simulink model "UAV_sync_known_sim"  (R2018b)
settings: Solver=ode23tb  StartTime=0.0  StopTime=35
values from neighbouring files (symbols this model uses):
  C_rho = 1.225    [SC42120_UAV_Preconditions.m]
  D0 = [M0 0 0 0 0 0 ... (first row only)    [SC42120_UAV_Preconditions.m]
  D1 = [eye(3)*M1 zeros(3,3) ... (first row only)    [UAV_sync_known.m]    (also in UAV_sync_unknown.m; UAV_sync_unknown_gap.m)
  Derivative_gain_phi = 50    [SC42120_UAV_Preconditions.m]
  Derivative_gain_psi = 50    [SC42120_UAV_Preconditions.m]
  Derivative_gain_theta = 50    [SC42120_UAV_Preconditions.m]
  Derivative_gain_x = 50    [SC42120_UAV_Preconditions.m]
  Derivative_gain_y = 50    [SC42120_UAV_Preconditions.m]
  Derivative_gain_z = 50    [SC42120_UAV_Preconditions.m]
  G = 9.80665    [SC42120_UAV_Preconditions.m]
  g0 = [0;0;-M0*G;0;0;0]    [SC42120_UAV_Preconditions.m]
  g1 = [0;0;-M1*G;0;0;0]    [UAV_sync_known.m]    (also in UAV_sync_unknown.m; UAV_sync_unknown_gap.m)
  I0 = [0.02 0 -0.01 ... (first row only)    [SC42120_UAV_Preconditions.m]
  I1 = [0.1 0 -0.01 ... (first row only)    [UAV_sync_known.m]    (also in UAV_sync_unknown.m; UAV_sync_unknown_gap.m)
  InitWind = [0;0;0]    [SC42120_UAV_Preconditions.m]
  Kp = diag(P)    [SC42120_UAV_Preconditions.m]
  Kv = diag(V)    [SC42120_UAV_Preconditions.m]
  M0 = 10    [SC42120_UAV_Preconditions.m]
  M1 = 20    [UAV_sync_known.m]    (also in UAV_sync_unknown.m; UAV_sync_unknown_gap.m)
  Proportional_phi = 50    [SC42120_UAV_Preconditions.m]
  Proportional_psi = 50    [SC42120_UAV_Preconditions.m]
  Proportional_theta = 50    [SC42120_UAV_Preconditions.m]
  Proportional_x = 50    [SC42120_UAV_Preconditions.m]
  Proportional_y = 50    [SC42120_UAV_Preconditions.m]
  Proportional_z = 50    [SC42120_UAV_Preconditions.m]
undefined symbols (not defined in the file or in its folder): Aero, APlane, Bxl, C, Ctr, deg, DiscIntNeverNeededParam, F, Guid, Init, Light, MIL, Path, rad, s, Trim, Utility
libraries: aerolibconvert2 x37, simulink x15, dspsigops x7, aerolibasang x6, shared6dof x3, simulink_extras x3, sharedutil x2, aerolibadyn x1, aerolibtransform2 x1, aerolibwind2 x1
(part 3 of 6)

== system UAV_sync_known_sim/Node 0/VF Approach/AUTOPILOT/Low-level Controllers/Pitch controller ==
  PitchReference : Inport  Unit=deg
  EulerAngles : Inport  Port=2  Unit=deg
  AngularRates : Inport  Port=3  Unit=deg/s
  Scaler : Inport  Port=4
  1/Ctr.Roll.RLL2SRV_TCONST : Gain  Gain=1/Ctr.Roll.RLL2SRV_TCONST
  Angle Conversion1 : aerolibconvert2/Angle Conversion  IU=deg  OU=rad
  Angle Conversion5 : aerolibconvert2/Angle Conversion  IU=deg  OU=rad
  Coordination offset : Subsystem
  Pitch PID : Subsystem
  Rate limiter : Saturate  UpperLimit=Ctr.Pitch.PTCH2SRV_RMAX_UP  LowerLimit=-Ctr.Pitch.PTCH2SRV_RMAX_DN  LinearizeAsGain=off
  Saturation1 : Saturate  UpperLimit=80  LowerLimit=-80
  Selector1 : Selector  InputPortWidth=3  IndexOptions=Index vector (dialog)  Indices=2  OutputSizes=1
  Selector2 : Selector  InputPortWidth=3  IndexOptions=Index vector (dialog)  Indices=1  OutputSizes=1
  Selector3 : Selector  InputPortWidth=3  IndexOptions=Index vector (dialog)  Indices=1  OutputSizes=1
  Selector4 : Selector  InputPortWidth=3  IndexOptions=Index vector (dialog)  Indices=2  OutputSizes=1
  Sum : Sum  Inputs=++|
  Sum1 : Sum  Inputs=|+-
  TRASH : Subsystem  Commented=on
  ElevDemand : Outport
  wires:
  AngularRates/1 -> Selector1/1
  Selector2/1 -> Angle Conversion1/1  "roll_angle"
  EulerAngles/1 -> Selector3/1, Selector2/1, Selector4/1
  Selector1/1 -> Pitch PID/3(Meas_pitch_rate)  "pitch_rate"
  Selector4/1 -> Sum1/2, [pitch_ang]
  PitchReference/1 -> Sum1/1
  Sum/1 -> Pitch PID/1(DesRate)
  Selector3/1 -> Pitch PID/4(Meas_roll_angle)
  Scaler/1 -> Pitch PID/2(Scaler)
  Coordination offset/1(Pitch_rate_correction) -> Sum/1
  Sum1/1 -> 1/Ctr.Roll.RLL2SRV_TCONST/1
  1/Ctr.Roll.RLL2SRV_TCONST/1 -> Rate limiter/1
  Rate limiter/1 -> Sum/2
  [pitch_ang] -> Angle Conversion5/1
  Saturation1/1 -> Coordination offset/2(bank)
  [Va] -> Coordination offset/3(Va)
  Angle Conversion5/1 -> Coordination offset/1(pitch)
  Angle Conversion1/1 -> Saturation1/1
  Pitch PID/1(ElevDemand) -> ElevDemand/1

== system UAV_sync_known_sim/Node 0/VF Approach/AUTOPILOT/Low-level Controllers/Roll controller ==
  RollReference : Inport  Unit=deg
  Euler angles : Inport  Port=2  Unit=deg
  AngularRates : Inport  Port=3  Unit=deg/s
  Scaler : Inport  Port=4
  Discrete PID Controller : simulink/Continuous/PID Controller  Controller=PI  Form=Parallel  TimeDomain=Discrete-time  SampleTime=Ctr.TS  IntegratorMethod=Forward Euler  FilterMethod=Forward Euler  ControllerParametersSource=internal  P=1.28067056525733  I=0.869761866515897  D=0  UseFilter=on  N=100  TunerSelectOption=Transfer Function Based (PID Tuner App)  InitialConditionSource=internal  InitialConditionForIntegrator=0  InitialConditionForFilter=0  DifferentiatorICPrevScaledInput=0  ExternalReset=none  TrackingMode=off  Kt=1  LimitOutput=on  UpperSaturationLimit=Ctr.Roll.RLL2SRV_RMAX  LowerSaturationLimit=-Ctr.Roll.RLL2SRV_RMAX  LinearizeAsGain=off  AntiWindupMode=clamping  Kb=1  POutMin=[]  POutMax=[]  IOutMin=[]  IOutMax=[]  DOutMin=[]  DOutMax=[]  NOutMin=[]  NOutMax=[]  SumOutMin=[]  SumOutMax=[]  SaturationOutMin=[]  SaturationOutMax=[]  PParamMin=[]  PParamMax=[]  IParamMin=[]  IParamMax=[]  DParamMin=[]  DParamMax=[]  NParamMin=[]  NParamMax=[]  KbParamMin=[]  KbParamMax=[]  KtParamMin=[]  KtParamMax=[]  KbOutMin=[]  KbOutMax=[]  KtOutMin=[]  KtOutMax=[]  IntegratorOutMin=[]  IntegratorOutMax=[]  FilterOutMin=[]  FilterOutMax=[]  SumI1OutMin=[]  SumI1OutMax=[]  SumI2OutMin=[]  SumI2OutMax=[]  SumI3OutMin=[]  SumI3OutMax=[]  SumI4OutMin=[]  SumI4OutMax=[]  SumDOutMin=[]  SumDOutMax=[]  DifferentiatorOutMin=[]  DifferentiatorOutMax=[]  FilterDiffOutCoefMin=[]  FilterDiffOutCoefMax=[]  ReciprocalOutMin=[]  ReciprocalOutMax=[]  SumDenOutMin=[]  SumDenOutMax=[]  SumNumOutMin=[]  SumNumOutMax=[]  DivideOutMin=[]  DivideOutMax=[]  IntegratorContinuousStateAttributes=''  IntegratorStateMustResolveToSignalObject=off  IntegratorRTWStateStorageClass=Auto  FilterContinuousStateAttributes=''  FilterStateMustResolveToSignalObject=off  FilterRTWStateStorageClass=Auto  ParallelPVariant=InternalParameters  IdealPVariant=Disabled  IVariant=InternalParameters  DVariant=Disabled  IntegratorVariant=Discrete  SatVariant=Enabled  AWVariant=DiscClampingParallel  PCopyVariant=Disabled  TRVariant=Disabled  FdbkBlocksVariant=Forward  IdealPFdbkVariant=Disabled  SatFdbkVariant=Disabled  DerivativeFilterVariant=Disabled  NVariant=Disabled  NCopyVariant=Disabled_SignalSpec  FilterICVariant=Disabled  IntegratorICVariant=InternalICs  ExternalResetVariant=Disabled  TRSumVariant=Passthrough  SumFdbkVariant=Disabled  SumVariant=Sum_PI
  Manual Switch : ManualSwitch  CurrentSetting=0
  Manual Switch1 : ManualSwitch
  OMEGA : Gain  Gain=Ctr.Roll.OMEGA
  Roll Rate Controller : Subsystem
  Roll Rate Controller (simpl. continuous) : Subsystem  Commented=on
  "Scaler " : InportShadow  Port=4
  Scope : Scope  NumInputPorts=2
  Scope1 : Scope
  Selector : Selector  InputPortWidth=3  IndexOptions=Index vector (dialog)  Indices=1  OutputSizes=1
  Selector1 : Selector  InputPortWidth=3  IndexOptions=Index vector (dialog)  Indices=1  OutputSizes=1
  Sum : Sum  Inputs=|+-
  gainsrmax(deg/s) : Saturate  UpperLimit=Ctr.Roll.RLL2SRV_RMAX  LowerLimit=-Ctr.Roll.RLL2SRV_RMAX
  AilDemand : Outport  Unit=deg
  wires:
  RollReference/1 -> Scope/1, Sum/1
  Scaler/1 -> Roll Rate Controller/3(Scaler)  "m/s"
  AngularRates/1 -> Selector1/1
  Euler angles/1 -> Selector/1
  Sum/1 -> OMEGA/1, Discrete PID Controller/1, Scope1/1
  Selector1/1 -> Roll Rate Controller (simpl. continuous)/2(Roll rate), Roll Rate Controller/2(Roll Rate)  "roll_rate"
  Selector/1 -> Scope/2, Sum/2
  Manual Switch/1 -> Roll Rate Controller (simpl. continuous)/1(Roll Rate Error), Roll Rate Controller/1(Desidered rate)  "roll_rate_erorr [deg/s]"
  Manual Switch1/1 -> AilDemand/1
  Roll Rate Controller/1(Ail_dem) -> Manual Switch1/1
  "Scaler "/1 -> Roll Rate Controller (simpl. continuous)/3(Scaler)  "m/s"
  Roll Rate Controller (simpl. continuous)/1(AilDemand) -> Manual Switch1/2
  OMEGA/1 -> gainsrmax(deg/s)/1
  gainsrmax(deg/s)/1 -> Manual Switch/2  "roll_rate_erorr [deg/s]"
  Discrete PID Controller/1 -> Manual Switch/1

== system UAV_sync_known_sim/Node 0/VF Approach/AUTOPILOT/Low-level Controllers/Side-slip angle controller ==
  note: - Ctr.Yaw.YAW2SRV_SLIP enables side-slip angle control (disabled)
      | - Ctr.Yaw.YAW2SRV_DAMP enables the yaw angle damping (enabled)
  note: Roll Mixer = Aileron Rudder Interconnect (ARI). Disabled cause it creates an additional roll-yaw cross-coupling.
  note: Roll mixer
  Yaw_rate : Inport
  "Euler angles " : Inport  Port=2
  accel_y : Inport  Port=3
  Scaler : Inport  Port=4
  AilDemand : Inport  Port=5
  Angle Conversion : aerolibconvert2/Angle Conversion  IU=rad  OU=deg
  Coordination offset : Subsystem
  "Ctr.Yaw.KFF_RDDRMIX " : Gain  Gain=-1*Ctr.Yaw.KFF_RDDRMIX
  Ctr.Yaw.YAW2SRV_DAMP : Gain  Gain=Ctr.Yaw.YAW2SRV_DAMP
  Ctr.Yaw.YAW2SRV_INT : Gain  Gain=Ctr.Yaw.YAW2SRV_INT
  Ctr.Yaw.YAW2SRV_SLIP : Gain  Gain=Ctr.Yaw.YAW2SRV_SLIP+0.25
  Discrete-Time Integrator : DiscreteIntegrator  SampleTime=Ctr.TS  UpperSaturationLimit=deg2rad(15)  LowerSaturationLimit=deg2rad(-15)  ICPrevOutput=DiscIntNeverNeededParam  ICPrevScaledInput=DiscIntNeverNeededParam
  Gain4 : Gain  Gain=-1
  High-Pass Filter : Subsystem
  Math Function : Math  Operator=square  SaturateOnIntegerOverflow=on
  Product : Product
  Saturation : Saturate  UpperLimit=45  LowerLimit=-45
  Scope : Scope
  Scope1 : Scope
  Scope2 : Scope
  Selector1 : Selector  InputPortWidth=3  IndexOptions=Index vector (dialog)  Indices=1  OutputSizes=1
  Selector4 : Selector  InputPortWidth=3  IndexOptions=Index vector (dialog)  Indices=2  OutputSizes=1
  Selector5 : Selector  InputPortWidth=3  IndexOptions=Index vector (dialog)  Indices=3  OutputSizes=1
  Sum : Sum  Inputs=|+-
  Sum1 : Sum  Inputs=|+-
  Sum2 : Sum  Inputs=|+-
  Sum3 : Sum  Inputs=|++
  on/off : Gain
  RudderDemand : Outport
  wires:
  Ctr.Yaw.YAW2SRV_SLIP/1 -> Sum/1
  Yaw_rate/1 -> Selector5/1
  Sum1/1 -> High-Pass Filter/1(In)  "r_err"
  High-Pass Filter/1(Out) -> Scope2/1, Sum2/2, Sum/2
  Sum/1 -> Ctr.Yaw.YAW2SRV_INT/1
  Ctr.Yaw.YAW2SRV_INT/1 -> Discrete-Time Integrator/1
  Discrete-Time Integrator/1 -> Sum2/1
  Sum2/1 -> Ctr.Yaw.YAW2SRV_DAMP/1
  Ctr.Yaw.YAW2SRV_DAMP/1 -> Product/1
  Scaler/1 -> Math Function/1
  Math Function/1 -> Product/2
  Product/1 -> Gain4/1
  Selector5/1 -> Sum1/1
  Angle Conversion/1 -> Sum3/1
  Gain4/1 -> Angle Conversion/1
  Sum3/1 -> Saturation/1
  "Ctr.Yaw.KFF_RDDRMIX "/1 -> Sum3/2
  Saturation/1 -> on/off/1
  AilDemand/1 -> "Ctr.Yaw.KFF_RDDRMIX "/1
  "Euler angles "/1 -> Selector1/1
  Coordination offset/1(yaw_rate_correction) -> Sum1/2
  Selector1/1 -> Coordination offset/1(Bank)
  accel_y/1 -> Selector4/1
  Selector4/1 -> Ctr.Yaw.YAW2SRV_SLIP/1, Scope/1
  on/off/1 -> RudderDemand/1, Scope1/1

== system UAV_sync_known_sim/Node 0/VF Approach/AUTOPILOT/Navigation Controller/PID ==
  err : Inport
  scaler : Inport  Port=2
  20Hz filter : DiscreteTransferFcn  Numerator=Ctr.Hdg2Roll.lowpass.num  Denominator=Ctr.Hdg2Roll.lowpass.den  SampleTime=Ctr.TS
  Constant9 : Constant  Value=Ctr.TS
  Digital Clock : DigitalClock  SampleTime=Ctr.TS
  Discrete Transfer Fcn : DiscreteTransferFcn  Numerator=[1 -1]  Denominator=[Ctr.TS 0]  SampleTime=Ctr.TS
  Discrete Transfer Fcn1 : DiscreteTransferFcn  Numerator=Ctr.TS  Denominator=[1 -1]  SampleTime=Ctr.TS
  Discrete Transfer Fcn2 : DiscreteTransferFcn  Numerator=1  Denominator=[1 -1]  SampleTime=Ctr.TS
  Goto : Goto  Commented=on  GotoTag=deltaT
  IMAX : Saturate  UpperLimit=Ctr.Hdg2Roll.IMAX  LowerLimit=-Ctr.Hdg2Roll.IMAX
  K_D : Gain  Commented=on  Gain=Ctr.Hdg2Roll.NAV_ROLL_D
  K_I : Gain  Gain=Ctr.Hdg2Roll.NAV_ROLL_I
  K_I1 : Gain  Gain=Ctr.Hdg2Roll.NAV_ROLL_I
  K_P : Gain  Gain=Ctr.Hdg2Roll.NAV_ROLL_P
  Manual Switch : ManualSwitch  CurrentSetting=0
  Product : Product
  Product2 : Product  Inputs=**
  Product3 : Product  Commented=on  Inputs=*/
  Product4 : Product
  Product5 : Product
  Scope : Scope  NumInputPorts=3
  Scope1 : Scope
  Scope2 : Scope  NumInputPorts=2
  Sum1 : Sum  Inputs=+++
  Sum3 : Sum  Commented=on  Inputs=|+-
  Sum4 : Sum  Inputs=|+-
  Unit Delay : UnitDelay  SampleTime=-1
  Unit Delay2 : UnitDelay  Commented=on  SampleTime=-1
  out : Outport
  wires:
  K_P/1 -> Product5/1
  err/1 -> Product/2, K_P/1, K_D/1, K_I/1
  IMAX/1 -> Scope/2, Sum1/2
  K_I/1 -> Discrete Transfer Fcn1/1
  Unit Delay/1 -> Sum4/2
  Digital Clock/1 -> Unit Delay/1, Sum4/1
  Manual Switch/1 -> Goto/1
  Constant9/1 -> Manual Switch/1
  Product2/1 -> IMAX/1
  20Hz filter/1 -> Product4/2
  Product4/1 -> Scope/3, Sum1/3
  Product5/1 -> Scope/1, Sum1/1
  Discrete Transfer Fcn1/1 -> Scope2/2, Product2/1
  scaler/1 -> Product2/2, Product5/2, Product4/1
  Sum1/1 -> out/1, Scope1/1
  K_D/1 -> Discrete Transfer Fcn/1
  Unit Delay2/1 -> Sum3/2
  Sum3/1 -> Product3/1
  Discrete Transfer Fcn/1 -> 20Hz filter/1
  Sum4/1 -> Product/1, Manual Switch/2
  K_I1/1 -> Discrete Transfer Fcn2/1
  Discrete Transfer Fcn2/1 -> Scope2/1
  Product/1 -> K_I1/1

== system UAV_sync_known_sim/Node 0/VF Approach/AUTOPILOT/Navigation Controller/Unwrap ==
  In : Inport
  Degrees to Radians : simulink_extras/Transformations/Degrees to Radians
  Radians to Degrees : simulink_extras/Transformations/Radians to Degrees
  Unwrap2 : dspsigops/Unwrap  tol=pi  InputProcessing=Columns as channels (frame based)  running=off
  Out : Outport
  wires:
  Unwrap2/1 -> Radians to Degrees/1
  In/1 -> Degrees to Radians/1
  Degrees to Radians/1 -> Unwrap2/1
  Radians to Degrees/1 -> Out/1

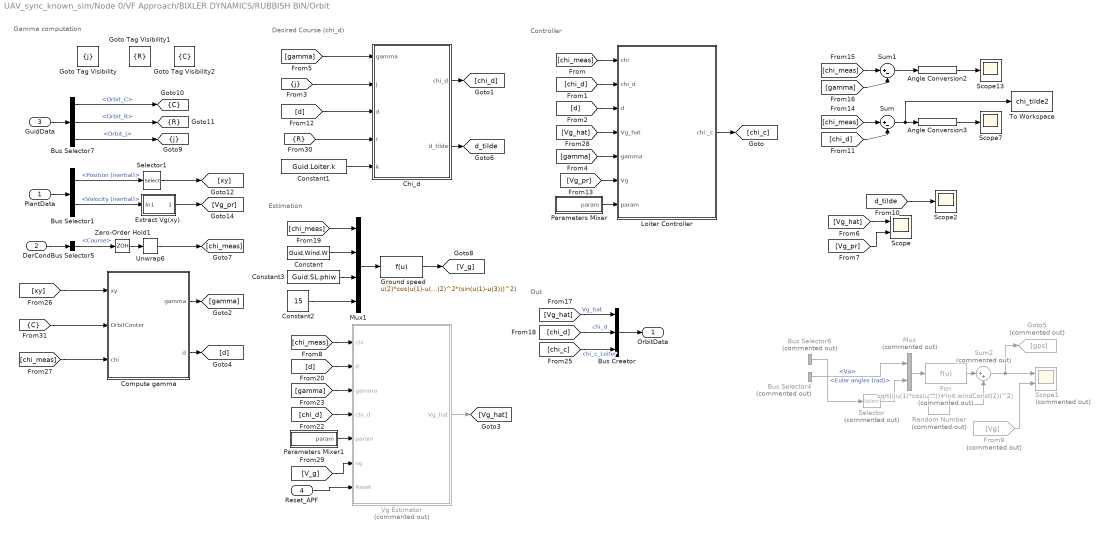
== system UAV_sync_known_sim/Node 0/VF Approach/BIXLER DYNAMICS/RUBBISH BIN/Orbit ==
  note: Out
  note: Controller
  note: Desired Course (chi_d)
  note: Gamma computation
  note: Estimation
  PlantData : Inport
  DerCond : Inport  Port=2
  GuidData : Inport  Port=3
  Reset_APF : Inport  Port=4
  Angle Conversion2 : aerolibconvert2/Angle Conversion  IU=rad  OU=deg
  Angle Conversion3 : aerolibconvert2/Angle Conversion  IU=rad  OU=deg
  Bus Creator : BusCreator  Inputs=3
  Bus Selector1 : BusSelector  OutputSignals=Position (inertial),Velocity (inertial)
  Bus Selector4 : BusSelector  Commented=on  OutputSignals=Va
  Bus Selector5 : BusSelector  OutputSignals=Course
  Bus Selector6 : BusSelector  Commented=on  OutputSignals=Euler angles (rad)
  Bus Selector7 : BusSelector  OutputSignals=Orbit_C,Orbit_R,Orbit_j
  Chi_d : Subsystem
  Compute gamma : Subsystem
  Constant : Constant  Value=Guid.Wind.W
  Constant1 : Constant  Value=Guid.Loiter.k
  Constant2 : Constant  Value=15
  Constant3 : Constant  Value=Guid.SL.phiw
  Extract Vg(xy). : Subsystem
  Fcn : Fcn  Commented=on  Expr=sqrt(( u(1)*cos(u(2))+Init.windConst(1) )^2 + (u(1)*sin(u(2))+Init.windConst(2))^2)
  From9 : From  Commented=on  GotoTag=Vg
  Goto Tag Visibility : GotoTagVisibility  GotoTag=j
  Goto Tag Visibility1 : GotoTagVisibility  GotoTag=R
  Goto Tag Visibility2 : GotoTagVisibility  GotoTag=C
  Goto5 : Goto  Commented=on  GotoTag=gps
  Ground speed : Fcn  Expr=u(2)*cos(u(1)-u(3))+sqrt(u(4)^2-u(2)^2*(sin(u(1)-u(3)))^2)
  Loiter Controller : Subsystem
  Mux : Mux  Commented=on  Inputs=2
  Mux1 : Mux
  Parameters Mixer : Subsystem
  Parameters Mixer1 : Subsystem
  Random Number : RandomNumber  Commented=on  Variance=0.05^2  SampleTime=0.2
  Scope : Scope  NumInputPorts=2
  Scope1 : Scope  Commented=on  NumInputPorts=2
  Scope13 : Scope
  Scope2 : Scope
  Scope7 : Scope
  Selector : Selector  Commented=on  InputPortWidth=3  IndexOptions=Index vector (dialog)  Indices=3  OutputSizes=1
  Selector1 : Selector  InputPortWidth=3  IndexOptions=Index vector (dialog)  Indices=[1 2]  OutputSizes=1
  Sum : Sum  Inputs=|+-
  Sum1 : Sum  Inputs=|+-
  Sum2 : Sum  Commented=on  Inputs=|++
  To Workspace : ToWorkspace  VariableName=chi_tilde2  SaveFormat=Timeseries  SampleTime=-1
  Unwrap6 : dspsigops/Unwrap  tol=pi  running=off
  Vg Estimator : Subsystem  Commented=on
  Zero-Order Hold1 : ZeroOrderHold  SampleTime=-1
  OrbitData : Outport
  tag scope: C=scoped, R=scoped, d_tilde=global, j=scoped
  wires:
  Compute gamma/1(gamma) -> [gamma]
  [Vg_hat] -> Bus Creator/1  "Vg_hat"
  [chi_d] -> Bus Creator/2  "chi_d"
  Bus Creator/1 -> OrbitData/1
  [chi_c] -> Bus Creator/3  "chi_c_Loiter"
  Bus Selector1/1 -> Selector1/1  "<Position (inertial)>"
  Selector1/1 -> [xy]
  Bus Selector1/2 -> Extract Vg(xy)./1(In1)  "<Velocity (inertial)>"
  Extract Vg(xy)./1(Out1) -> [Vg_pr]
  [chi_meas] -> Sum/1
  [chi_d] -> Sum/2
  Sum/1 -> To Workspace/1, Angle Conversion3/1
  [chi_meas] -> Sum1/1
  [gamma] -> Sum1/2
  Sum1/1 -> Angle Conversion2/1
  Angle Conversion2/1 -> Scope13/1
  Angle Conversion3/1 -> Scope7/1
  Compute gamma/2(d) -> [d]
  [xy] -> Compute gamma/1(xy)
  [chi_meas] -> Compute gamma/3(chi)
  [gamma] -> Chi_d/1(gamma)
  [j] -> Chi_d/2(j)
  [d] -> Chi_d/3(d)
  [R] -> Chi_d/4(r)
  Constant1/1 -> Chi_d/5(k)
  Chi_d/1(chi_d) -> [chi_d]
  Chi_d/2(d_tilde) -> [d_tilde]
  [chi_meas] -> Vg Estimator/1(chi)
  [d] -> Vg Estimator/2(d)
  [gamma] -> Vg Estimator/3(gamma)
  [chi_d] -> Vg Estimator/4(chi_d)
  Parameters Mixer1/1(param) -> Vg Estimator/5(param)
  Vg Estimator/1(Vg_hat) -> [Vg_hat]
  [chi_meas] -> Loiter Controller/1(chi)
  [chi_d] -> Loiter Controller/2(chi_d)
  [d] -> Loiter Controller/3(d)
  [Vg_hat] -> Loiter Controller/4(Vg_hat)
  [gamma] -> Loiter Controller/5(gamma)
  Loiter Controller/1(chi:_c) -> [chi_c]
  Parameters Mixer/1(param) -> Loiter Controller/7(param)
  DerCond/1 -> Bus Selector5/1
  Zero-Order Hold1/1 -> Unwrap6/1
  Unwrap6/1 -> [chi_meas]
  [C] -> Compute gamma/2(OrbitCenter)
  [Vg_hat] -> Scope/1
  [Vg_pr] -> Scope/2
  [d_tilde] -> Scope2/1
  Bus Selector4/1 -> Mux/1  "<Va>"
  Bus Selector6/1 -> Selector/1  "<Euler angles (rad)>"
  Selector/1 -> Mux/2
  Mux/1 -> Fcn/1
  Fcn/1 -> Sum2/1
  Random Number/1 -> Sum2/2
  Sum2/1 -> Goto5/1, Scope1/1
  From9/1 -> Scope1/2
  PlantData/1 -> Bus Selector1/1
  Bus Selector5/1 -> Zero-Order Hold1/1  "<Course>"
  [Vg_pr] -> Loiter Controller/6(Vg)
  [chi_meas] -> Mux1/1
  Constant/1 -> Mux1/2
  Constant3/1 -> Mux1/3
  Constant2/1 -> Mux1/4
  Mux1/1 -> Ground speed/1
  [V_g] -> Vg Estimator/6(vg)
  Ground speed/1 -> [V_g]
  GuidData/1 -> Bus Selector7/1
  Bus Selector7/3 -> [j]  "<Orbit_j>"
  Bus Selector7/2 -> [R]  "<Orbit_R>"
  Bus Selector7/1 -> [C]  "<Orbit_C>"
  Reset_APF/1 -> Vg Estimator/7(Reset)

== system UAV_sync_known_sim/Node 0/VF Approach/BIXLER DYNAMICS/RUBBISH BIN/Reference Signals ==
  Throttle : Inport
  Bus Creator : BusCreator  Inputs='Roll Reference (rad)','Pitch Reference (rad)','Yaw Reference (rad)'
  Pitch Reference Generator : Subsystem
  Roll Reference Generator : Subsystem
  Yaw Reference Generator : Subsystem
  ActuatorsReference : Outport
  wires:
  Roll Reference Generator/1(RollDemand) -> Bus Creator/1  "Roll Reference (rad)"
  Yaw Reference Generator/1(YawDemand) -> Bus Creator/3  "Yaw Reference (rad)"
  Pitch Reference Generator/1(Pitch Reference) -> Bus Creator/2  "Pitch Reference (rad)"
  Bus Creator/1 -> ActuatorsReference/1
  Throttle/1 -> Pitch Reference Generator/1(Throttle)

== system UAV_sync_known_sim/Node 0/VF Approach/BIXLER DYNAMICS/RUBBISH BIN/Reference Signals1 ==
  Throttle : Inport
  Bus Creator : BusCreator  Inputs='Roll Reference (rad)','Pitch Reference (rad)','Yaw Reference (rad)'
  Pitch Reference Generator : Subsystem
  Roll Reference Generator : Subsystem
  Yaw Reference Generator : Subsystem
  ActuatorsReference : Outport
  wires:
  Throttle/1 -> Pitch Reference Generator/1(Throttle)
  Bus Creator/1 -> ActuatorsReference/1
  Pitch Reference Generator/1(Pitch Reference) -> Bus Creator/2  "Pitch Reference (rad)"
  Yaw Reference Generator/1(YawDemand) -> Bus Creator/3  "Yaw Reference (rad)"
  Roll Reference Generator/1(RollDemand) -> Bus Creator/1  "Roll Reference (rad)"

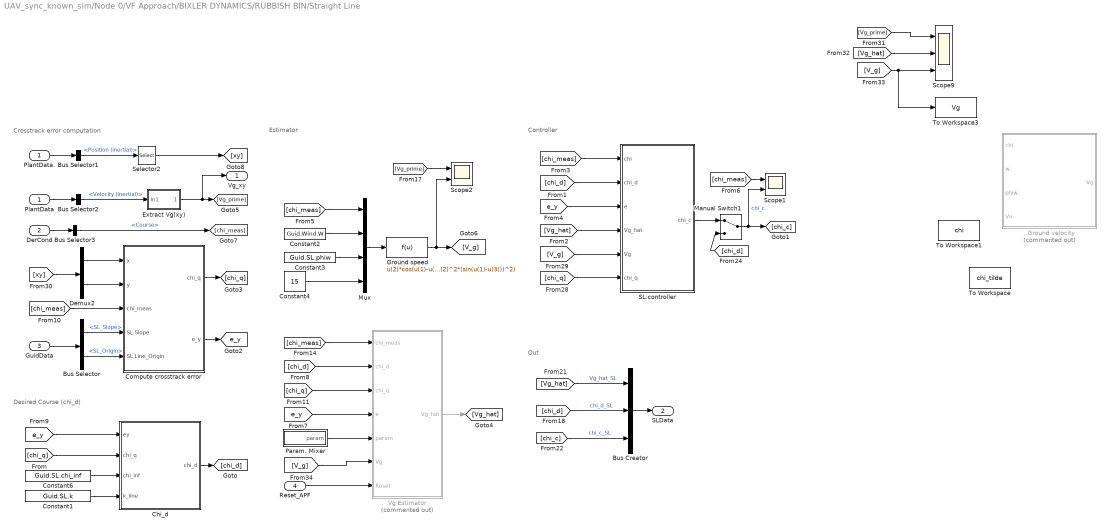
== system UAV_sync_known_sim/Node 0/VF Approach/BIXLER DYNAMICS/RUBBISH BIN/Straight Line ==
  note: Out
  note: Controller
  note: Estimator
  note: Desired Course (chi_d)
  note: Crosstrack error computation
  PlantData : Inport
  DerCond : Inport  Port=2
  GuidData : Inport  Port=3
  Reset_APF : Inport  Port=4
  ..Ground velocity : MATLAB Function  Commented=on  TreatAsAtomicUnit=on
  Bus Creator : BusCreator  Inputs=3
  Bus Selector : BusSelector  OutputSignals=SL_Slope,SL_Origin
  Bus Selector1 : BusSelector  OutputSignals=Position (inertial)
  Bus Selector2 : BusSelector  OutputSignals=Velocity (inertial)
  Bus Selector3 : BusSelector  OutputSignals=Course
  Chi_d : Subsystem
  Compute crosstrack error : Subsystem
  Constant1 : Constant  Value=Guid.SL.k
  Constant2 : Constant  Value=Guid.Wind.W
  Constant3 : Constant  Value=Guid.SL.phiw
  Constant4 : Constant  Value=15
  Constant6 : Constant  Value=Guid.SL.chi_inf
  Demux2 : Demux  Outputs=2
  Extract Vg(xy) : Subsystem
  Ground speed : Fcn  Expr=u(2)*cos(u(1)-u(3))+sqrt(u(4)^2-u(2)^2*(sin(u(1)-u(3)))^2)
  Manual Switch1 : ManualSwitch
  Mux : Mux
  Param. Mixer : Subsystem
  PlantData. : InportShadow
  SL.controller : Subsystem
  Scope1 : Scope  NumInputPorts=2
  Scope2 : Scope  NumInputPorts=2
  Scope9 : Scope  NumInputPorts=3
  Selector2 : Selector  InputPortWidth=3  IndexOptions=Index vector (dialog)  Indices=[1 2]  OutputSizes=1
  To Workspace : ToWorkspace  VariableName=chi_tilde  SaveFormat=Timeseries  SampleTime=-1
  To Workspace1 : ToWorkspace  VariableName=chi  SaveFormat=Timeseries  SampleTime=-1
  To Workspace3 : ToWorkspace  VariableName=Vg  SaveFormat=Timeseries  SampleTime=-1
  Vg Estimator : Subsystem  Commented=on
  Vg_xy : Outport
  SLData : Outport  Port=2
  tag scope: e_y=global
  wires:
  Compute crosstrack error/2(e_y) -> [e_y]
  Compute crosstrack error/1(chi_q) -> [chi_q]
  [chi_meas] -> Compute crosstrack error/3(chi_meas)
  [chi_meas] -> SL.controller/1(chi)
  Demux2/1 -> Compute crosstrack error/1(x)
  Demux2/2 -> Compute crosstrack error/2(y)
  DerCond/1 -> Bus Selector3/1
  [chi_d] -> Manual Switch1/2
  Bus Selector/2 -> Compute crosstrack error/5(SL.Line_Origin)  "<SL_Origin>"
  [e_y] -> Chi_d/1(ey)
  [chi_q] -> Chi_d/2(chi_q)
  Constant6/1 -> Chi_d/3(chi_inf)
  Constant1/1 -> Chi_d/4(k_line)
  Chi_d/1(chi_d) -> [chi_d]
  [chi_d] -> SL.controller/2(chi_d)
  [e_y] -> SL.controller/3(e)
  [Vg_hat] -> SL.controller/4(Vg_hat)
  [chi_q] -> SL.controller/6(chi_q)
  SL.controller/1(chi_c) -> Manual Switch1/1
  [chi_meas] -> Scope1/1
  GuidData/1 -> Bus Selector/1
  Bus Selector/1 -> Compute crosstrack error/4(SL.Slope)  "<SL_Slope>"
  Manual Switch1/1 -> [chi_c], Scope1/2  "chi_c"
  [chi_d] -> Bus Creator/2  "chi_d_SL"
  [Vg_hat] -> Bus Creator/1  "Vg_hat_SL"
  [chi_c] -> Bus Creator/3  "chi_c_SL"
  Extract Vg(xy)/1(Out1) -> Vg_xy/1, [Vg_prime]
  Bus Creator/1 -> SLData/1
  PlantData/1 -> Bus Selector2/1
  Bus Selector2/1 -> Extract Vg(xy)/1(In1)  "<Velocity (inertial)>"
  Bus Selector3/1 -> [chi_meas]  "<Course>"
  PlantData./1 -> Bus Selector1/1
  Bus Selector1/1 -> Selector2/1  "<Position (inertial)>"
  Selector2/1 -> [xy]
  [xy] -> Demux2/1
  [chi_meas] -> Vg Estimator/1(chi_meas)
  [chi_d] -> Vg Estimator/2(chi_d)
  [chi_q] -> Vg Estimator/3(chi_q)
  [e_y] -> Vg Estimator/4(e)
  Param. Mixer/1(param) -> Vg Estimator/5(param)
  Vg Estimator/1(Vg_hat) -> [Vg_hat]
  [V_g] -> SL.controller/5(Vg)
  [chi_meas] -> Mux/1
  Constant2/1 -> Mux/2
  Constant3/1 -> Mux/3
  Ground speed/1 -> Scope2/2, [V_g]
  [Vg_prime] -> Scope2/1
  [Vg_prime] -> Scope9/1
  [Vg_hat] -> Scope9/2
  [V_g] -> To Workspace3/1, Scope9/3
  Constant4/1 -> Mux/4
  [V_g] -> Vg Estimator/6(Vg)
  Mux/1 -> Ground speed/1
  Reset_APF/1 -> Vg Estimator/7(Reset)

== system UAV_sync_known_sim/Node 0/VF Approach/BIXLER DYNAMICS/RUBBISH BIN/TECS ==
  PlantData : Inport
  TAS_dem : Inport  Port=2  Unit=m/s
  HeightDemand : Inport  Port=3  Unit=m
  Bus Selector : BusSelector  OutputSignals=SPE_dem,SPE_weighting,SKE_dem,SKE_weighting,SPEdot_dem,SKEdot_dem,SPE_est,SKE_est,SPEdot,SKEdot
  Bus Selector1 : BusSelector  OutputSignals=SKE_dem,SPE_dem,SPE_est,SKE_est,SKEdot,SPEdot,SKEdot_dem,SPEdot_dem
  Energy Balance : Subsystem
  Energy calculations : Subsystem
  Gain : Gain
  PITCH : Subsystem
  PITCH1 : Subsystem
  PlantData1 : InportShadow
  Scope1 : Scope
  THROTTLE : Subsystem
  THROTTLE1 : Subsystem
  Zero-Order Hold : ZeroOrderHold  SampleTime=Ctr.TECS.TS
  Zero-Order Hold1 : ZeroOrderHold  SampleTime=Ctr.TECS.TS
  Zero-Order Hold2 : ZeroOrderHold  SampleTime=Ctr.TECS.TS
  ThrottleReference : Outport  Unit=%
  PitchReference : Outport  Port=2  Unit=deg
  wires:
  PlantData/1 -> Zero-Order Hold/1
  TAS_dem/1 -> Zero-Order Hold1/1
  HeightDemand/1 -> Zero-Order Hold2/1
  PITCH/1(Pitch) -> PitchReference/1
  THROTTLE/1(ThrottleReference) -> Gain/1
  PlantData1/1 -> THROTTLE1/9(PlantData), THROTTLE/9(PlantData)
  Gain/1 -> Scope1/1, ThrottleReference/1
  Energy calculations/1(EnergyBus) -> Bus Selector1/1, Bus Selector/1
  Energy Balance/1(SEB_error) -> PITCH1/1(SEB_error), PITCH/1(SEB_error)
  Energy Balance/2(SEBdot_dem) -> PITCH1/2(SEBdot_dem), PITCH/2(SEBdot_dem)
  Energy Balance/3(SEBdot_error) -> PITCH1/3(SEBdot_error), PITCH/3(SEBdot_error)
  Bus Selector/10 -> Energy Balance/10(SKEdot_est)  "<SKEdot>"
  Bus Selector/9 -> Energy Balance/9(SPEdot_est)  "<SPEdot>"
  Bus Selector/8 -> Energy Balance/8(SKE_est)  "<SKE_est>"
  Bus Selector/7 -> Energy Balance/7(SPE_est)  "<SPE_est>"
  Bus Selector/6 -> Energy Balance/6(SKEdot_dem)  "<SKEdot_dem>"
  Bus Selector/5 -> Energy Balance/5(SPEdot_dem)  "<SPEdot_dem>"
  Bus Selector/4 -> Energy Balance/4(SKE_weighting)  "<SKE_weighting>"
  Bus Selector/3 -> Energy Balance/3(SKE_dem)  "<SKE_dem>"
  Bus Selector/2 -> Energy Balance/2(SPE_weighting)  "<SPE_weighting>"
  Bus Selector/1 -> Energy Balance/1(SPE_dem)  "<SPE_dem>"
  Bus Selector1/1 -> THROTTLE1/1(SKE_dem), THROTTLE/1(SKE_dem)  "<SKE_dem>"
  Bus Selector1/2 -> THROTTLE1/2(SPE_dem), THROTTLE/2(SPE_dem)  "<SPE_dem>"
  Bus Selector1/3 -> THROTTLE1/3(SPE_est), THROTTLE/3(SPE_est)  "<SPE_est>"
  Bus Selector1/4 -> THROTTLE/4(SKE_est), THROTTLE1/4(SKE_est)  "<SKE_est>"
  Bus Selector1/5 -> THROTTLE1/5(SKEdot), THROTTLE/5(SKEdot)  "<SKEdot>"
  Bus Selector1/6 -> THROTTLE1/6(SPEdot), THROTTLE/6(SPEdot)  "<SPEdot>"
  Bus Selector1/7 -> THROTTLE1/7(SKEdot_dem), THROTTLE/7(SKEdot_dem)  "<SKEdot_dem>"
  Bus Selector1/8 -> THROTTLE1/8(SPEdot_dem), THROTTLE/8(SPEdot_dem)  "<SPEdot_dem>"
  Zero-Order Hold/1 -> Energy calculations/1(PlantData)
  Zero-Order Hold1/1 -> Energy calculations/2(TAS_dem)
  Zero-Order Hold2/1 -> Energy calculations/3(HeightDemand)

== system UAV_sync_known_sim/Node 0/VF Approach/BIXLER DYNAMICS/Vehicle Airframe/Aerodynamics ==
  PlantData : Inport
  DerCond : Inport  Port=2
  Control : Inport  Port=3
  Aerodynamic Coefficients : Subsystem
  Bus Selector : BusSelector  OutputSignals=Va,alpha,beta
  ControlIncrements : Subsystem
  Demux : Demux  Outputs=6
  "DerCond " : InportShadow  Port=2
  Forces/Moments : Subsystem
  Goto Tag Visibility : GotoTagVisibility  GotoTag=alphaRad
  Sum{2..9} (8 alike) : Sum  Inputs=|++
  AeroForces : Outport  Unit=N
  AeroMoments : Outport  Port=2  Unit=N*m
  wires:
  Aerodynamic Coefficients/1(Coeff) -> Demux/1
  Sum7/1 -> Forces/Moments/2(Cy)
  Sum8/1 -> Forces/Moments/4(Cl)
  ControlIncrements/6(Cy_rudd) -> Sum7/2
  Forces/Moments/1(Fxyz) -> AeroForces/1
  ControlIncrements/3(CD_elev) -> Sum5/2
  Sum5/1 -> Forces/Moments/1(CD)
  ControlIncrements/8(Cn_rudd) -> Sum9/2
  Sum6/1 -> Forces/Moments/3(CL)
  ControlIncrements/7(Cl_rudd) -> Sum8/2
  Demux/1 -> Sum5/1
  Demux/3 -> Sum6/1
  Demux/2 -> Sum7/1
  Demux/5 -> Sum4/1
  Sum3/1 -> Sum8/1
  Demux/4 -> Sum3/1
  ControlIncrements/2(Cl_ail) -> Sum3/2
  Sum2/1 -> Sum9/1
  ControlIncrements/1(Cn_ail) -> Sum2/2
  ControlIncrements/4(CL_elev) -> Sum6/2
  Sum4/1 -> Forces/Moments/5(Cm)
  ControlIncrements/5(Cm_elev) -> Sum4/2
  Demux/6 -> Sum2/1
  Sum9/1 -> Forces/Moments/6(Cn)
  DerCond/1 -> ControlIncrements/1(DerCond), Bus Selector/1
  Control/1 -> ControlIncrements/2(Control)
  PlantData/1 -> Aerodynamic Coefficients/1(PlantData)
  Forces/Moments/2(Mlmn) -> AeroMoments/1
  Bus Selector/2 -> Aerodynamic Coefficients/3(alpha(rad))  "<alpha>"
  Bus Selector/3 -> Aerodynamic Coefficients/4(beta(rad))  "<beta>"
  "DerCond "/1 -> Forces/Moments/7(DerCond)
  Bus Selector/1 -> Aerodynamic Coefficients/2(Va)  "<Va>"

== system UAV_sync_known_sim/Node 0/VF Approach/BIXLER DYNAMICS/Vehicle Airframe/Gravity Force ==
  PlantData : Inport
  Bus Selector : BusSelector  OutputSignals=From inertial to body matrix
  Constant : Constant  Value=Bxl.mass
  Constant1 : Constant  Value=0
  Constant2 : Constant  Value=0
  Gain : Gain  Gain=C.g
  Mux : Mux  Inputs=3
  Product : Product  Multiplication=Matrix(*)
  Fg : Outport  Unit=N
  wires:
  Constant2/1 -> Mux/2
  Constant/1 -> Gain/1
  Constant1/1 -> Mux/1
  Gain/1 -> Mux/3
  PlantData/1 -> Bus Selector/1
  Bus Selector/1 -> Product/1  "<From inertial to body matrix>"
  Mux/1 -> Product/2
  Product/1 -> Fg/1

== system UAV_sync_known_sim/Node 0/VF Approach/BIXLER DYNAMICS/Vehicle Airframe/Propulsion ==
  note: For the sign convention (nose down)
  note: (this was designed to push down the aircraft, because of the high lift force generated when increasing the throttle)
  Throttle : Inport
  DerCond : Inport  Port=2
  By interpolation : Subsystem
  Degrees to Radians : simulink_extras/Transformations/Degrees to Radians
  Gain : Gain  Gain=Bxl.propDist
  Gain2 : Gain  Gain=-1
  Manual Switch : ManualSwitch
  Motor mount angle(deg) : Constant  Value=10
  Mux : Mux  Inputs=3
  Mux1 : Mux  Inputs=3
  Mux2 : Mux  Inputs=2
  Mux3 : Mux  Inputs=2
  Propeller model (Bernoulli) : Subsystem
  T_x : Fcn  Expr=u(1)*cos(u(2))
  T_z : Fcn  Expr=u(1)*sin(u(2))
  Thrust_Y : Constant  Value=0
  Thrust_l : Constant  Value=0
  Thrust_n : Constant  Value=0
  F : Outport  Unit=N
  M : Outport  Port=2  Unit=N*m
  wires:
  Manual Switch/1 -> Gain2/1, Mux3/1, Mux2/1
  Thrust_n/1 -> Mux1/3
  Thrust_Y/1 -> Mux/2
  Motor mount angle(deg)/1 -> Degrees to Radians/1
  Degrees to Radians/1 -> Mux2/2, Mux3/2
  Gain/1 -> Mux1/2  "Thrust_m"
  Gain2/1 -> Gain/1
  Thrust_l/1 -> Mux1/1
  Throttle/1 -> By interpolation/1(In1), Propeller model (Bernoulli)/2(Throttle)
  DerCond/1 -> Propeller model (Bernoulli)/1(DerCond)
  Propeller model (Bernoulli)/1(Thrust) -> Manual Switch/1
  Mux/1 -> F/1
  Mux1/1 -> M/1
  T_z/1 -> Mux/3
  T_x/1 -> Mux/1
  Mux2/1 -> T_x/1
  Mux3/1 -> T_z/1
  By interpolation/1(Out1) -> Manual Switch/2

== system UAV_sync_known_sim/Node 0/VF Approach/BIXLER DYNAMICS/Vehicle Airframe/to Omega_e ==
  euler : Inport
  ome_b : Inport  Port=2
  MATLAB Function : MATLAB Function  TreatAsAtomicUnit=on
  ome_e : Outport
  wires:
  MATLAB Function/1(omega_e) -> ome_e/1
  euler/1 -> MATLAB Function/1(attitude)
  ome_b/1 -> MATLAB Function/2(omega_b)

== system UAV_sync_known_sim/Node 0/VF Approach/PATH FOLLOWING/Orbit Path Following (Enabled Subsystem)/Chi_d ==
  gamma : Inport
  j : Inport  Port=2
  d : Inport  Port=3
  r : Inport  Port=4
  Bias : Bias  Bias=-2*pi
  Constant1 : Constant  Value=Guid.Loiter.k
  Manual Switch : ManualSwitch
  Mux : Mux  Inputs=5
  While Iterator Subsystem : Subsystem  Commented=on  TreatAsAtomicUnit=on
  While Iterator Subsystem2 : Subsystem  Commented=on  TreatAsAtomicUnit=on
  chi_d calc. : Fcn  Expr=u(1) + u(2)*(pi/2 + atan(u(5)*(u(3)-u(4))))
  d_tilde calc. : Fcn  Expr=u(3)-u(4)
  chi_d : Outport
  d_tilde : Outport  Port=2
  wires:
  gamma/1 -> Mux/1
  Constant1/1 -> Mux/5
  d/1 -> Mux/3
  r/1 -> Mux/4
  j/1 -> Mux/2
  Mux/1 -> chi_d calc./1, d_tilde calc./1
  While Iterator Subsystem/1(gaooa_out) -> While Iterator Subsystem2/3(IC), While Iterator Subsystem2/1(gamma)
  d_tilde calc./1 -> d_tilde/1
  chi_d calc./1 -> Bias/1, Manual Switch/1
  Manual Switch/1 -> chi_d/1
  Bias/1 -> Manual Switch/2

== system UAV_sync_known_sim/Node 0/VF Approach/PATH FOLLOWING/Orbit Path Following (Enabled Subsystem)/Compute gamma and distance to center ==
  xy : Inport
  OrbitCenter : Inport  Port=2
  chi : Inport  Port=3
  L.PolarCoord : MATLAB Function  Commented=on  TreatAsAtomicUnit=on
  MATLAB Function : MATLAB Function  TreatAsAtomicUnit=on
  Mux : Mux  Inputs=2
  Unwrap : dspsigops/Unwrap  Commented=through  tol=pi  InputProcessing=Columns as channels (frame based)  running=off
  Zero-Order Hold2 : ZeroOrderHold  SampleTime=-1
  Zero-Order Hold4 : ZeroOrderHold  SampleTime=-1
  Zero-Order Hold5 : ZeroOrderHold  Commented=on  SampleTime=-1
  distance calc. : Fcn  Expr=sqrt((u(1)-u(3))^2+(u(2)-u(4))^2)
  gamma calc. : Fcn  Expr=atan2(u(2)-u(4),u(1)-u(3))
  gamma : Outport
  d : Outport  Port=2
  wires:
  OrbitCenter/1 -> Zero-Order Hold4/1
  distance calc./1 -> d/1
  gamma calc./1 -> Unwrap/1
  xy/1 -> Zero-Order Hold2/1
  Zero-Order Hold2/1 -> Mux/1
  Mux/1 -> distance calc./1, gamma calc./1
  Zero-Order Hold4/1 -> Mux/2
  chi/1 -> MATLAB Function/2(chi)
  Unwrap/1 -> MATLAB Function/1("gamma ")
  MATLAB Function/1(gamma) -> gamma/1

== system UAV_sync_known_sim/Node 0/VF Approach/PATH FOLLOWING/Orbit Path Following (Enabled Subsystem)/Loiter Controller ==
  chi : Inport
  chi_d : Inport  Port=2
  d : Inport  Port=3
  Vg_hat : Inport  Port=4
  gamma : Inport  Port=5
  Vg : Inport  Port=6
  Constant2 : Constant  Value=Guid.Method
  Loiter Controller : MATLAB Function  TreatAsAtomicUnit=on
  Multiport Switch : MultiPortSwitch  DataPortOrder=Zero-based contiguous  DataPortIndices={1,2,9}  zeroidx=on
  Parameters Mixer : Subsystem
  chi_c : Outport
  wires:
  chi_d/1 -> Loiter Controller/2(chi_d)
  d/1 -> Loiter Controller/3(d)
  Vg_hat/1 -> Multiport Switch/2
  chi/1 -> Loiter Controller/1(chi)
  Parameters Mixer/1(param) -> Loiter Controller/6(param)
  gamma/1 -> Loiter Controller/5(gamma)
  Loiter Controller/1(y) -> chi_c/1
  Multiport Switch/1 -> Loiter Controller/4(Vg)
  [Vg_prime] -> Multiport Switch/4
  Constant2/1 -> Multiport Switch/1
  Vg/1 -> Multiport Switch/3

== system UAV_sync_known_sim/Node 0/VF Approach/PATH FOLLOWING/Orbit Path Following (Enabled Subsystem)/Vg Estimator ==
  chi : Inport
  d : Inport  Port=2
  gamma : Inport  Port=3
  chi_d : Inport  Port=4
  vg : Inport  Port=5
  DerCond : Inport  Port=6
  Bus Selector1 : BusSelector  OutputSignals=Va
  "Estimator " : MATLAB Function  TreatAsAtomicUnit=on
  Integrator1 : Integrator  InitialConditionSource=external  InitialCondition=Guid.Vg0  LimitOutput=on  UpperSaturationLimit=Guid.EstMax  LowerSaturationLimit=0
  Parameters Mixer : Subsystem
  Vg_hat : Outport
  wires:
  chi_d/1 -> "Estimator "/4(chi_d)
  Integrator1/1 -> Vg_hat/1, "Estimator "/7(Vg_hat)  "Vg_hat"
  d/1 -> "Estimator "/2(d)
  chi/1 -> "Estimator "/1(chi)
  gamma/1 -> "Estimator "/3(gamma)
  vg/1 -> [Vg], "Estimator "/6(Vg)
  Parameters Mixer/1(param) -> "Estimator "/5(param)
  DerCond/1 -> Bus Selector1/1
  Bus Selector1/1 -> Parameters Mixer/1(airspeed)  "<Va>"
  [Vg] -> Integrator1/2
  "Estimator "/1(Vg2_hat_dot) -> Integrator1/1

== system UAV_sync_known_sim/Node 0/VF Approach/PATH FOLLOWING/Straight-line Path Following (Enabled Subsystem)/Chi_d ==
  ey : Inport
  chi_q : Inport  Port=2
  chi_inf : Inport  Port=3
  k_line : Inport  Port=4
  Mux : Mux
  Vector Field (straight line) : MATLAB Function  Commented=on  TreatAsAtomicUnit=on
  chi_d calc. : Fcn  Expr=u(2) - 1*u(3)*2/pi*atan(u(4)*u(1))
  chi_d : Outport
  wires:
  chi_inf/1 -> Mux/3
  k_line/1 -> Mux/4
  ey/1 -> Mux/1
  chi_q/1 -> Mux/2
  Mux/1 -> chi_d calc./1
  chi_d calc./1 -> chi_d/1

== system UAV_sync_known_sim/Node 0/VF Approach/PATH FOLLOWING/Straight-line Path Following (Enabled Subsystem)/Compute crosstrack error ==
  xy : Inport
  SL.Slope : Inport  Port=2
  SL.Line_Origin : Inport  Port=3
  chi : Inport  Port=4
  Mux : Mux  Inputs=3
  Unwrap : dspsigops/Unwrap  Commented=through  tol=pi  InputProcessing=Columns as channels (frame based)  running=off
  chi_q calc. : Fcn  Expr=atan2(u(2),u(1))
  chi_q_correction : MATLAB Function  TreatAsAtomicUnit=on
  e_y calc. : Fcn  Expr=-sin(u(1))*(u(2)-u(4)) + cos(u(1))*(u(3)-u(5))
  chi_q : Outport
  e_y : Outport  Port=2  Unit=m
  wires:
  xy/1 -> Mux/2
  e_y calc./1 -> e_y/1
  SL.Line_Origin/1 -> Mux/3
  chi_q calc./1 -> chi_q_correction/1("chi_q ")
  Unwrap/1 -> Mux/1, chi_q/1
  SL.Slope/1 -> chi_q calc./1
  Mux/1 -> e_y calc./1
  chi_q_correction/1(chi_q) -> Unwrap/1
  chi/1 -> chi_q_correction/2(chi)

== system UAV_sync_known_sim/Node 0/VF Approach/PATH FOLLOWING/Straight-line Path Following (Enabled Subsystem)/SL.controller ==
  chi : Inport  Unit=rad
  chi_d : Inport  Port=2  Unit=rad
  e : Inport  Port=3
  Vg_hat : Inport  Port=4  Unit=m/s
  Vg : Inport  Port=5  Unit=m/s
  chi_q : Inport  Port=6  Unit=rad
  Constant2 : Constant  Value=Guid.Method
  Multiport Switch : MultiPortSwitch  DataPortOrder=Zero-based contiguous  DataPortIndices={1,2,9}  zeroidx=on
  Param. Mixer : Subsystem
  SL.Controller : MATLAB Function  TreatAsAtomicUnit=on
  chi_c : Outport
  wires:
  Param. Mixer/1(param) -> SL.Controller/5(param)
  Multiport Switch/1 -> SL.Controller/4(Vg)
  chi/1 -> SL.Controller/1(chi)
  chi_d/1 -> SL.Controller/2(chi_d)
  e/1 -> SL.Controller/3(e)
  chi_q/1 -> SL.Controller/6(chi_q)
  [Vg_prime] -> Multiport Switch/4
  SL.Controller/1(chi_c) -> chi_c/1
  Constant2/1 -> Multiport Switch/1
  Vg/1 -> Multiport Switch/3
  Vg_hat/1 -> Multiport Switch/2

== system UAV_sync_known_sim/Node 0/VF Approach/PATH FOLLOWING/Straight-line Path Following (Enabled Subsystem)/Vg Estimator ==
  chi_meas : Inport
  chi_d : Inport  Port=2
  chi_q : Inport  Port=3
  e : Inport  Port=4
  Vg : Inport  Port=5
  DerCond : Inport  Port=6
  Bus Selector1 : BusSelector  OutputSignals=Va
  Integrator : Integrator  InitialConditionSource=external  InitialCondition=Guid.Vg0  LimitOutput=on  UpperSaturationLimit=Guid.EstMax  LowerSaturationLimit=0  IgnoreLimit=on
  Param. Mixer : Subsystem
  SL_Estimator : MATLAB Function  TreatAsAtomicUnit=on
  Vg_hat : Outport
  wires:
  Param. Mixer/1(param) -> SL_Estimator/5(param)
  chi_meas/1 -> SL_Estimator/1(chi)
  chi_q/1 -> SL_Estimator/3(chi_q)
  e/1 -> SL_Estimator/4(e)
  SL_Estimator/1(Vg_hat_dot) -> Integrator/1
  Integrator/1 -> SL_Estimator/7(Vg_hat), Vg_hat/1  "Vg2_hat"
  chi_d/1 -> SL_Estimator/2(chi_d)
  Vg/1 -> [Vg], SL_Estimator/6(Vg)
  DerCond/1 -> Bus Selector1/1
  Bus Selector1/1 -> Param. Mixer/1(Va)  "<Va>"
  [Vg] -> Integrator/2

== system UAV_sync_known_sim/Node 1/Node 1/Inverse Dynamics Control/Inverse Dynamic 1/Inner Controller ==
  e_x : Inport
  e_y : Inport  Port=2
  e_z : Inport  Port=3
  e_phi : Inport  Port=4
  e_theta : Inport  Port=5
  e_psi : Inport  Port=6
  e_xdot : Inport  Port=7
  e_zdot : Inport  Port=8
  e_phidot : Inport  Port=9
  e_thetadot : Inport  Port=10
  e_psidot : Inport  Port=11
  e_ydot : Inport  Port=12
  Add{1..6} (6 alike) : Sum
  Constant1 : Constant  Value=Derivative_gain_x
  Constant10 : Constant  Value=Proportional_theta
  Constant11 : Constant  Value=Proportional_psi
  Constant12 : Constant  Value=Derivative_gain_psi
  Constant2 : Constant  Value=Derivative_gain_y
  Constant3 : Constant  Value=Proportional_y
  Constant4 : Constant  Value=Derivative_gain_z
  Constant5 : Constant  Value=Proportional_z
  Constant6 : Constant  Value=Derivative_gain_phi
  Constant7 : Constant  Value=Proportional_phi
  Constant8 : Constant  Value=Derivative_gain_theta
  Constant9 : Constant  Value=Proportional_x
  Product{1..12} (12 alike) : Product
  act1 : Outport
  act2 : Outport  Port=2
  act3 : Outport  Port=3
  act4 : Outport  Port=4
  act5 : Outport  Port=5
  act6 : Outport  Port=6
  wires:
  Add5/1 -> act5/1
  Add6/1 -> act6/1
  Add1/1 -> act1/1
  Add3/1 -> act3/1
  Product7/1 -> Add1/2
  Constant9/1 -> Product7/2
  Product1/1 -> Add1/1
  e_x/1 -> Product7/1
  e_xdot/1 -> Product1/2
  Constant1/1 -> Product1/1
  Product3/1 -> Add3/1
  Product9/1 -> Add3/2
  Constant5/1 -> Product9/2
  Constant4/1 -> Product3/1
  e_z/1 -> Product9/1
  Constant7/1 -> Product10/2
  e_phidot/1 -> Product4/2
  Constant6/1 -> Product4/1
  e_phi/1 -> Product10/1
  Product4/1 -> Add4/1
  Product11/1 -> Add5/1
  Constant10/1 -> Product5/2
  e_thetadot/1 -> Product11/2
  Constant8/1 -> Product11/1
  e_theta/1 -> Product5/1
  Product5/1 -> Add5/2
  Constant11/1 -> Product12/2
  Constant12/1 -> Product6/1
  e_psidot/1 -> Product6/2
  Product12/1 -> Add6/2
  e_psi/1 -> Product12/1
  Product6/1 -> Add6/1
  Product10/1 -> Add4/2
  e_zdot/1 -> Product3/2
  e_y/1 -> Product2/2
  Product2/1 -> Add2/1
  Product8/1 -> Add2/2
  Constant2/1 -> Product2/1
  e_ydot/1 -> Product8/1
  Constant3/1 -> Product8/2
  Add2/1 -> act2/1
  Add4/1 -> act4/1

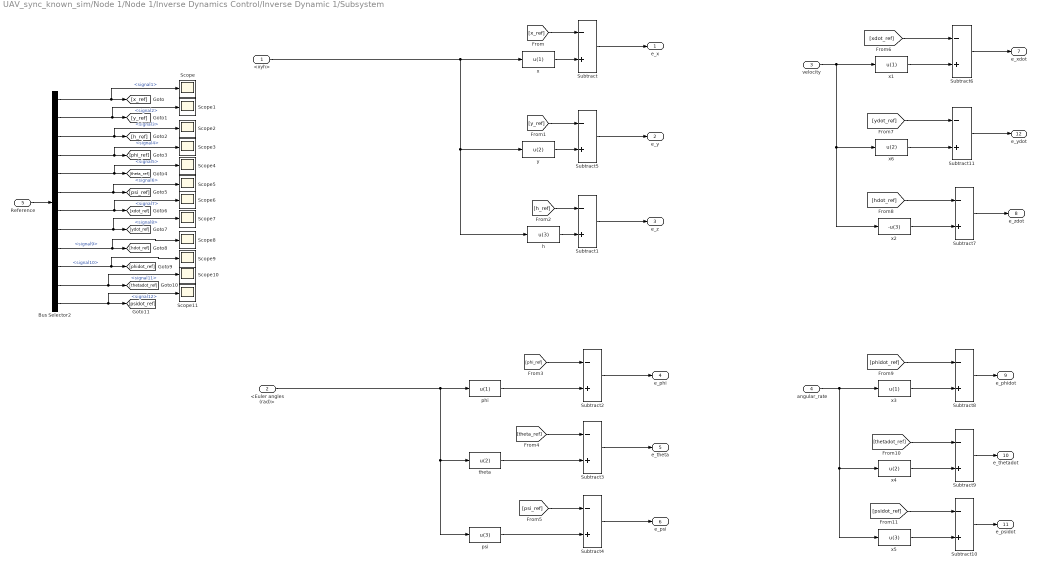
== system UAV_sync_known_sim/Node 1/Node 1/Inverse Dynamics Control/Inverse Dynamic 1/Subsystem ==
  <xyh> : Inport
  <Euler angles (rad)> : Inport  Port=2
  velocity : Inport  Port=3
  angular_rate : Inport  Port=4
  Reference : Inport  Port=5
  Bus Selector2 : BusSelector  OutputSignals=signal1,signal2,signal3,signal4,signal5,signal6,signal7,signal8,signal9,signal10,signal11,signal12
  Scope{,1..11} (12 alike) : Scope
  Subtract{,1..11} (12 alike) : Sum  Inputs=-+
  h : Fcn  Expr=u(3)
  phi : Fcn  Expr=u(1)
  psi : Fcn  Expr=u(3)
  theta : Fcn  Expr=u(2)
  x : Fcn  Expr=u(1)
  x1 : Fcn  Expr=u(1)
  x2 : Fcn  Expr=-u(3)
  x3 : Fcn  Expr=u(1)
  x4 : Fcn  Expr=u(2)
  x5 : Fcn  Expr=u(3)
  x6 : Fcn  Expr=u(2)
  y : Fcn  Expr=u(2)
  e_x : Outport
  e_y : Outport  Port=2
  e_z : Outport  Port=3
  e_phi : Outport  Port=4
  e_theta : Outport  Port=5
  e_psi : Outport  Port=6
  e_xdot : Outport  Port=7
  e_zdot : Outport  Port=8
  e_phidot : Outport  Port=9
  e_thetadot : Outport  Port=10
  e_psidot : Outport  Port=11
  e_ydot : Outport  Port=12
  wires:
  [h_ref] -> Subtract1/1
  h/1 -> Subtract1/2
  <Euler angles (rad)>/1 -> psi/1, theta/1, phi/1
  <xyh>/1 -> h/1, y/1, x/1
  [x_ref] -> Subtract/1
  x/1 -> Subtract/2
  Subtract10/1 -> e_psidot/1
  Subtract9/1 -> e_thetadot/1
  Subtract6/1 -> e_xdot/1
  Subtract5/1 -> e_y/1
  y/1 -> Subtract5/2
  x2/1 -> Subtract7/2
  x1/1 -> Subtract6/2
  velocity/1 -> x6/1, x2/1, x1/1
  Subtract/1 -> e_x/1
  Subtract2/1 -> e_phi/1
  angular_rate/1 -> x3/1, x4/1, x5/1
  x4/1 -> Subtract9/2
  Subtract3/1 -> e_theta/1
  x5/1 -> Subtract10/2
  Subtract4/1 -> e_psi/1
  [xdot_ref] -> Subtract6/1
  [hdot_ref] -> Subtract7/1
  Subtract7/1 -> e_zdot/1
  Subtract8/1 -> e_phidot/1
  Subtract11/1 -> e_ydot/1
  [y_ref] -> Subtract5/1
  Subtract1/1 -> e_z/1
  [ydot_ref] -> Subtract11/1
  x6/1 -> Subtract11/2
  [phidot_ref] -> Subtract8/1
  [thetadot_ref] -> Subtract9/1
  [psidot_ref] -> Subtract10/1
  phi/1 -> Subtract2/2
  x3/1 -> Subtract8/2
  Reference/1 -> Bus Selector2/1
  Bus Selector2/1 -> Scope/1, [x_ref]  "<signal1>"
  Bus Selector2/2 -> Scope1/1, [y_ref]  "<signal2>"
  Bus Selector2/3 -> Scope2/1, [h_ref]  "<signal3>"
  Bus Selector2/4 -> Scope3/1, [phi_ref]  "<signal4>"
  Bus Selector2/5 -> Scope4/1, [theta_ref]  "<signal5>"
  Bus Selector2/6 -> Scope5/1, [psi_ref]  "<signal6>"
  Bus Selector2/7 -> Scope6/1, [xdot_ref]  "<signal7>"
  Bus Selector2/8 -> Scope7/1, [ydot_ref]  "<signal8>"
  Bus Selector2/9 -> Scope8/1, [hdot_ref]  "<signal9>"
  Bus Selector2/12 -> Scope11/1, [psidot_ref]  "<signal12>"
  Bus Selector2/10 -> Scope9/1, [phidot_ref]  "<signal10>"
  Bus Selector2/11 -> Scope10/1, [thetadot_ref]  "<signal11>"
  theta/1 -> Subtract3/2
  psi/1 -> Subtract4/2
  [phi_ref] -> Subtract2/1
  [theta_ref] -> Subtract3/1
  [psi_ref] -> Subtract4/1

== system UAV_sync_known_sim/Node 1/Node 1/Inverse Dynamics Control/Inverse Dynamic 2/Rot_Matrix [3x3] ==
  p : Inport
  q : Inport  Port=2
  r : Inport  Port=3
  Zero : Inport  Port=4
  I1 : Inport  Port=5
  I5 : Inport  Port=6
  I9 : Inport  Port=7
  I3_I7 : Inport  Port=8
  Add : Sum  Inputs=+-
  Add1 : Sum  Inputs=+-
  Gain1 : Gain  Gain=-1
  Gain2 : Gain  Gain=-1
  Gain3 : Gain  Gain=-1
  Product{1..5} (5 alike) : Product
  Reshape : Reshape  OutputDimensionality=Customize  OutputDimensions=[3,3]
  Vector Concatenate : Concatenate  NumInputs=9
  Out1 : Outport
  wires:
  Add/1 -> Gain1/1, Vector Concatenate/2
  Vector Concatenate/1 -> Reshape/1
  Gain3/1 -> Vector Concatenate/3
  Gain2/1 -> Vector Concatenate/8
  I1/1 -> Product3/2
  I9/1 -> Product4/2
  Product2/1 -> Gain3/1, Vector Concatenate/7
  I5/1 -> Product2/2
  Gain1/1 -> Vector Concatenate/4
  Add1/1 -> Vector Concatenate/6, Gain2/1
  r/1 -> Product5/1, Product4/1
  q/1 -> Product2/1
  Zero/1 -> Vector Concatenate/9, Vector Concatenate/5, Vector Concatenate/1
  Reshape/1 -> Out1/1
  p/1 -> Product1/1, Product3/1
  I3_I7/1 -> Product5/2, Product1/2
  Product4/1 -> Add/1
  Product1/1 -> Add/2
  Product5/1 -> Add1/2
  Product3/1 -> Add1/1

== system UAV_sync_known_sim/Node 1/Node 1/Inverse Dynamics Control/Inverse Dynamic 2/Trans_Matrix [3x3] ==
  p : Inport
  q : Inport  Port=2
  r : Inport  Port=3
  zero : Inport  Port=4
  M : Inport  Port=5
  Gain2 : Gain  Gain=-1
  Gain3 : Gain  Gain=-1
  Gain4 : Gain  Gain=-1
  Product2 : Product
  Product3 : Product
  Product4 : Product
  Reshape : Reshape  OutputDimensionality=Customize  OutputDimensions=[3,3]
  Vector Concatenate : Concatenate  NumInputs=9
  Out1 : Outport
  wires:
  r/1 -> Product2/1
  q/1 -> Product3/1
  Reshape/1 -> Out1/1
  Product2/1 -> Vector Concatenate/4, Gain4/1
  Vector Concatenate/1 -> Reshape/1
  Product4/1 -> Vector Concatenate/8, Gain2/1
  Gain2/1 -> Vector Concatenate/6
  p/1 -> Product4/1
  M/1 -> Product4/2, Product3/2, Product2/2
  Product3/1 -> Gain3/1, Vector Concatenate/3
  Gain3/1 -> Vector Concatenate/7
  zero/1 -> Vector Concatenate/5, Vector Concatenate/1, Vector Concatenate/9
  Gain4/1 -> Vector Concatenate/2

== system UAV_sync_known_sim/Node 0/VF Approach/AUTOPILOT/Low-level Controllers/Pitch controller/Coordination offset ==
  pitch : Inport  Unit=rad
  bank : Inport  Port=2  Unit=rad
  Va : Inport  Port=3  Unit=m/s
  Abs1 : Abs
  Angular Velocity Conversion : aerolibconvert2/Angular Velocity Conversion  IU=rad/s  OU=deg/s
      settings: SourceProductName=Aerospace Blockset
  Constant : Constant  Value=C.g
  Constant3 : Constant  Value=Ctr.Pitch.PTCH2SRV_RLL
  Product : Product  Inputs=***
  Product1 : Product  Inputs=*/**
  bank_1 : InportShadow  Port=2  Unit=rad
  cos : Subsystem
  sin : Subsystem
  tan : Subsystem
  Pitch_rate_correction : Outport
  wires:
  Product1/1 -> Abs1/1
  cos/1(Out1) -> Product/1
  tan/1(Out1) -> Product1/3
  sin/1(Out1) -> Product1/4
  bank/1 -> tan/1(In1)
  Va/1 -> Product1/2
  Product/1 -> Angular Velocity Conversion/1
  Constant3/1 -> Product/3
  Abs1/1 -> Product/2
  Constant/1 -> Product1/1
  pitch/1 -> cos/1(In1)
  bank_1/1 -> sin/1(In1)
  Angular Velocity Conversion/1 -> Pitch_rate_correction/1

== system UAV_sync_known_sim/Node 0/VF Approach/AUTOPILOT/Low-level Controllers/Pitch controller/Pitch PID ==
  DesRate : Inport  Unit=deg/s
  Scaler : Inport  Port=2
  Meas_pitch_rate : Inport  Port=3  Unit=deg/s
  Meas_roll_angle : Inport  Port=4
  +-45 : Saturate  UpperLimit=45  LowerLimit=-45
  Adjust integrator gain : Subsystem  Commented=on
  Anti-windup : Subsystem
  Constant1 : Constant  Value=Ctr.Pitch.K_P
  Constant10 : Constant  Value=0
  Constant11 : Constant  Value=APlane.EAS2TAS
  Constant12 : Constant  Value=Ctr.Pitch.PTCH2SRV_D
  Constant2 : Constant  Value=Ctr.Pitch.PTCH2SRV_FF
  Constant4 : Constant  Value=Ctr.Pitch.PTCH2SRV_I
  Constant7 : Constant  Value=APlane.EAS2TAS
  Constant9 : Constant  Value=Ctr.TS
  Ctr.Pitch.PTCH2SRV_TCONST2 : Gain  Gain=Ctr.Pitch.PTCH2SRV_TCONST
  Gain : Gain  Gain=-1
  Meas_pitch_rate_1 : InportShadow  Port=3  Unit=deg/s
  MinMax : MinMax  Function=max  Inputs=2
  Product : Product
  Product1 : Product  Inputs=****
  Product2 : Product  Inputs=*/
  Product3 : Product  Inputs=*/
  Product4 : Product  Inputs=***
  Product5 : Product  Inputs=***
  Product6 : Product  Inputs=***
  Scaler_{1..4} (4 alike) : InportShadow  Port=2
  Subsystem : Subsystem  Commented=on
  Sum : Sum  Inputs=|+-
  Sum1 : Sum  Inputs=++|
  Sum5 : Sum  Inputs=++++
  Unit Delay1 : UnitDelay  SampleTime=Ctr.TS
  Unit Delay2 : UnitDelay  SampleTime=Ctr.TS
  intLimScaled : Saturate  UpperLimit=Ctr.Roll.RLL2SRV_IMAX_SCALED  LowerLimit=-Ctr.Roll.RLL2SRV_IMAX_SCALED;
  ElevDemand : Outport
  wires:
  [rateErr] -> Product4/1
  Product4/1 -> Sum5/4  "PID_D"
  Product5/1 -> Sum5/2  "PID_P"
  Product6/1 -> Sum5/3  "PID_FF"
  Scaler_3/1 -> Product6/3
  [des_rate] -> Product6/2
  Anti-windup/1(y_int) -> Sum1/2
  Constant10/1 -> MinMax/2
  Product/1 -> Product1/1, [rateErr]  "rate error"
  Product1/1 -> Anti-windup/1(u)  "integrator_delta"
  Constant9/1 -> Product1/3
  Sum/1 -> Product/1
  Scaler/1 -> Product/2
  Scaler_1/1 -> Product1/4
  Constant2/1 -> Product3/1
  Constant1/1 -> MinMax/1
  Constant12/1 -> Product4/2
  Scaler_4/1 -> Product5/3
  Constant7/1 -> Product2/2
  MinMax/1 -> Product2/1
  Constant11/1 -> Product3/2
  Product3/1 -> Product6/1  "k_ff"
  Scaler_2/1 -> Product4/3
  [des_rate] -> Product5/2
  Product2/1 -> Product5/1  "kp_ff"
  Unit Delay2/1 -> Sum1/1
  Unit Delay1/1 -> Anti-windup/2(y)
  Sum1/1 -> intLimScaled/1
  intLimScaled/1 -> Unit Delay2/1, Sum5/1  "PID_I"
  [lastO] -> Unit Delay1/1
  Ctr.Pitch.PTCH2SRV_TCONST2/1 -> Product1/2
  DesRate/1 -> Sum/1, [des_rate]
  Meas_pitch_rate/1 -> Sum/2
  Constant4/1 -> Ctr.Pitch.PTCH2SRV_TCONST2/1
  Sum5/1 -> [lastO], +-45/1  "last_out"
  Gain/1 -> ElevDemand/1
  +-45/1 -> Gain/1
  Meas_roll_angle/1 -> Subsystem/2(Meas_roll_angle)
  Meas_pitch_rate_1/1 -> Subsystem/3(Meas_pitch_rate)
